simulink model "joystick"  (R2023a)
settings: Solver=VariableStepAuto  StartTime=0.0  StopTime=inf  RelTol=1e-3
libraries: dspnetwork x1
settings Model: Creator=Usuario  LastModifiedBy=Usuario
settings DataIOCC: LimitDataPoints=on  MaxDataPoints=25000

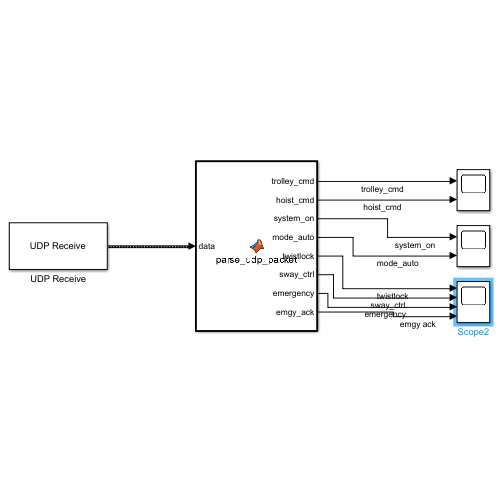
[thumbnail: Simulink's stored preview of the top-level diagram]
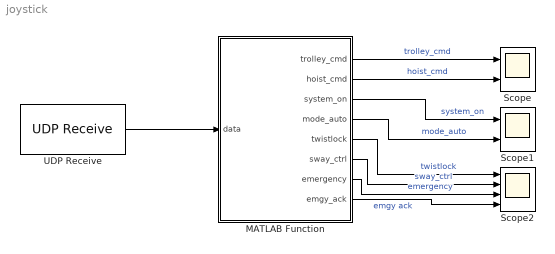
== system joystick ==
  MATLAB Function : MATLAB Function  TreatAsAtomicUnit=on
  Scope : Scope  NumInputPorts=2
  Scope1 : Scope  NumInputPorts=2
  Scope2 : Scope  NumInputPorts=4
  UDP Receive : dspnetwork/UDP Receive  localURL='0.0.0.0'  localPort=5005  remoteURL='0.0.0.0'  remotePort=-1  recvBufferSize=14  dims=255  signalDatatype=uint8  isComplex=off  isVarSize=on  showBlockingTime=off  blockingTime=0  sampletime=1  blockPlatform=[]
      settings: LibrarySourceBlock=dspsrcs4/UDP Receive
  wires:
  UDP Receive/1 -> MATLAB Function/1(data)
  MATLAB Function/1(trolley_cmd) -> Scope/1  "trolley_cmd"
  MATLAB Function/2(hoist_cmd) -> Scope/2  "hoist_cmd"
  MATLAB Function/3(system_on) -> Scope1/1  "system_on"
  MATLAB Function/4(mode_auto) -> Scope1/2  "mode_auto"
  MATLAB Function/5(twistlock) -> Scope2/1  "twistlock"
  MATLAB Function/6(sway_ctrl) -> Scope2/2  "sway_ctrl"
  MATLAB Function/7(emergency) -> Scope2/3  "emergency"
  MATLAB Function/8(emgy_ack) -> Scope2/4  "emgy ack"

== matlab function joystick/MATLAB Function ==
  data: trolley_cmd output; hoist_cmd output; system_on output; mode_auto output; twistlock output; sway_ctrl output; emergency output; emgy_ack output; data input
function [trolley_cmd, hoist_cmd, system_on, mode_auto, twistlock, sway_ctrl, emergency, emgy_ack] = parse_udp_packet(data)
% parse_udp_packet  Desempaqueta el datagrama de 14 bytes enviado por controller_reader.py
%
% Entrada:
%   data  : uint8(1x14) — bytes crudos del bloque UDP Receive
%
% Salidas (todas double):
%   trolley_cmd  [-4.0 .. +4.0] m/s   consigna velocidad carro
%   hoist_cmd    [-1.5 .. +1.5] m/s   consigna velocidad izaje
%   system_on    0/1   Sistema ON/OFF
%   mode_auto    0/1   0=Manual  1=Auto
%   twistlock    0/1   0=Abierto 1=Cerrado
%   sway_ctrl    0/1   Control de balanceo ON/OFF
%   emergency    0/1   Emergencia activa
%   emgy_ack     0/1   ACK de emergencia global
%
% Formato del paquete Python: struct.pack('!ffBBBBBB', ...)
%   Big-endian: bytes 1-4 float32, 5-8 float32, 9-14 uint8
% -----------------------------------------------------------------------

% Valores por defecto (paquete malformado o vacío)
trolley_cmd = 0;
hoist_cmd   = 0;
system_on   = 0;
mode_auto   = 0;
twistlock   = 0;
sway_ctrl   = 0;
emergency   = 0;
emgy_ack    = 0;

if numel(data) < 14
    return
end

raw = uint8(data(:)');   % forzar fila 1x14

% ── Floats big-endian → invertir bytes antes de typecast ──────────────
%    Python '!' = big-endian; x86/MATLAB = little-endian
trolley_cmd = double(typecast(raw(4:-1:1), 'single'));
hoist_cmd   = double(typecast(raw(8:-1:5), 'single'));

% ── Flags uint8 (un byte cada uno) ────────────────────────────────────
system_on = double(raw(9));
mode_auto = double(raw(10));
twistlock = double(raw(11));
sway_ctrl = double(raw(12));
emergency = double(raw(13));
emgy_ack  = double(raw(14));
